simulink model "ModelSupervisor2"  (R2014b)
settings: Solver=ode3  StartTime=0.0  StopTime=T_max  FixedStep=h  RelTol=1e-3
values from neighbouring files (symbols this model uses):
  b = 0.1    [Input_LQR.m]    (also in TestKalman.m; TestSuper.m; TestVahidComparison.m; parameter.m)
  g = 9.81    [Input_LQR.m]    (also in TestKalman.m; TestSuper.m; TestVahidComparison.m; parameter.m = 9.8)
  h = 0.01    [Input_LQR.m]    (also in TestKalman.m = 0.001; TestSuper.m = 0.001; TestVahidComparison.m = 0.001; parameter.m)
  k = 0.15    [Input_LQR.m]    (also in TestKalman.m; TestSuper.m; TestVahidComparison.m; parameter.m)
  L = 1.4    [Input_LQR.m]    (also in TestKalman.m; TestSuper.m = 1.025; TestVahidComparison.m)
  M = 1    [Input_LQR.m]    (also in TestKalman.m; TestSuper.m; TestVahidComparison.m; parameter.m)
  m = 3/4    (= 0.75)    [Input_LQR.m]    (also in TestKalman.m; TestSuper.m; TestVahidComparison.m; parameter.m)
  theta_0 = 0    [Input_LQR.m]    (also in TestKalman.m = 0.1; TestSuper.m = 0.1; TestVahidComparison.m = 0.1)
  theta_dot0 = 0    [Input_LQR.m]    (also in TestKalman.m; TestSuper.m; TestVahidComparison.m)
  x_0 = 0    [Input_LQR.m]    (also in TestKalman.m; TestSuper.m; TestVahidComparison.m)
  x_dot0 = 0    [Input_LQR.m]    (also in TestKalman.m; TestSuper.m; TestVahidComparison.m)
undefined symbols (not defined in the file or in its folder): A_kA2, B_kA2, C_kA2, D_kA2
libraries: simulink x4
settings Model: Creator=Erik  LastModifiedBy=Erik
settings SolverCC: AlgebraicLoopSolver=LineSearch
settings OptimizationCC: UseDivisionForNetSlopeComputation=off  SimCompilerOptimization=off
settings DebuggingCC: FrameProcessingCompatibilityMsg=error
settings RTWCC: RTWCompilerOptimization=off
settings ConfigComp: CovMetricSettings=dw  CovHtmlReporting=on  CovSaveCumulativeToWorkspaceVar=on  CovSaveSingleToWorkspaceVar=on  CovModelRefEnable=Off  CovExternalEMLEnable=off  CovSFcnEnable=off

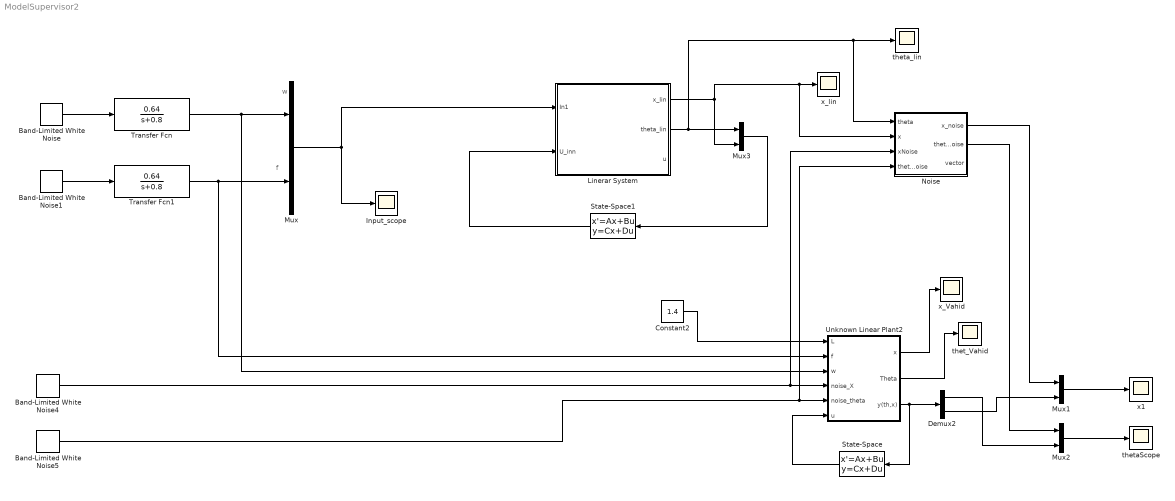
== system ModelSupervisor2 ==
  note: f
  note: w
  Band-Limited White Noise : simulink/Sources/Band-Limited White Noise  Cov=10  Ts=h  seed=[23343]
  Band-Limited White Noise1 : simulink/Sources/Band-Limited White Noise  Cov=10e-4  Ts=h  seed=[23344]
  Band-Limited White Noise4 : simulink/Sources/Band-Limited White Noise  Cov=10e-7  Ts=h  seed=[23343]
  Band-Limited White Noise5 : simulink/Sources/Band-Limited White Noise  Cov=10e-7  Ts=h  seed=[23344]
  Constant2 : Constant  Value=1.4
  Demux2 : Demux  Outputs=2
  Input_scope : Scope
      settings: YMin=-4  YMax=3  SaveName=ScopeData4
  Linerar System : Subsystem
  Mux{,1..3} (4 alike) : Mux  Inputs=2
  Noise : Subsystem
  State-Space : StateSpace  A=A_kA2  B=B_kA2  C=C_kA2  D=D_kA2  X0=0
  State-Space1 : StateSpace  A=A_kA2  B=B_kA2  C=C_kA2  D=D_kA2  X0=0
  Transfer Fcn : TransferFcn  Numerator=[0.64]  Denominator=[1 0.8]
  Transfer Fcn1 : TransferFcn  Numerator=[0.64]  Denominator=[1 0.8]
  Unknown Linear Plant2 : Subsystem
  thet_Vahid : Scope
      settings: SaveName=ScopeData3
  thetaScope : Scope
      settings: SaveName=ScopeData12
  theta_lin : Scope
      settings: YMin=-0.08  YMax=0.1  SaveName=ScopeData2
  x1 : Scope
      settings: YMin=-0.3  YMax=0.5  SaveName=ScopeData11
  x_Vahid : Scope
      settings: YMin=-0.15  YMax=0.1
  x_lin : Scope
      settings: YMin=-0.5  YMax=0.5
  wires:
  Mux/1 -> Linerar System/1(In1), Input_scope/1
  Band-Limited White Noise/1 -> Transfer Fcn/1
  Band-Limited White Noise1/1 -> Transfer Fcn1/1
  Linerar System/1(x_lin) -> Mux3/2, Noise/2(x), x_lin/1
  Unknown Linear Plant2/3(y(th,x)) -> Demux2/1, State-Space/1
  State-Space/1 -> Unknown Linear Plant2/6(u)
  Constant2/1 -> Unknown Linear Plant2/1(L)
  Demux2/1 -> Mux2/2
  Transfer Fcn/1 -> Mux/1, Unknown Linear Plant2/3(w)
  Transfer Fcn1/1 -> Unknown Linear Plant2/2(f), Mux/2
  Band-Limited White Noise4/1 -> Unknown Linear Plant2/4(noise_X), Noise/3(xNoise)
  Mux1/1 -> x1/1
  Mux2/1 -> thetaScope/1
  Linerar System/2(theta_lin) -> Mux3/1, Noise/1(theta), theta_lin/1
  Demux2/2 -> Mux1/2
  State-Space1/1 -> Linerar System/2(" U_inn")
  Mux3/1 -> State-Space1/1
  Noise/1(x_noise) -> Mux1/1
  Noise/2(theta_noise) -> Mux2/1
  Band-Limited White Noise5/1 -> Noise/4(thetaNoise), Unknown Linear Plant2/5(noise_theta)
  Unknown Linear Plant2/2(Theta) -> thet_Vahid/1
  Unknown Linear Plant2/1(x) -> x_Vahid/1

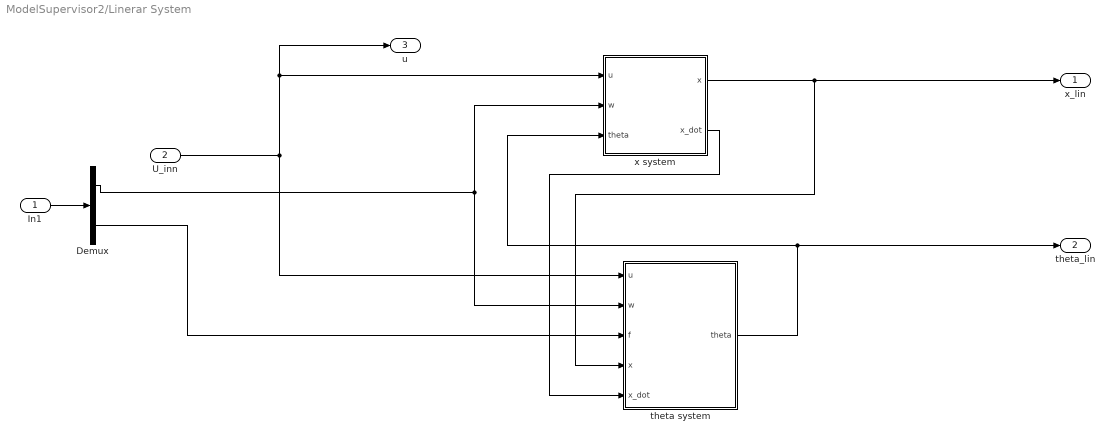
== system ModelSupervisor2/Linerar System ==
  In1 : Inport
  " U_inn" : Inport  Port=2
  Demux : Demux  Outputs=2
  "theta system " : Subsystem
  x system : Subsystem
  x_lin : Outport
  theta_lin : Outport  Port=2
  u : Outport  Port=3
  wires:
  x system/1(x) -> "theta system "/4(x), x_lin/1
  Demux/1 -> "theta system "/2(w), x system/2(w)
  "theta system "/1(theta) -> theta_lin/1, x system/3(theta)
  Demux/2 -> "theta system "/3(f)
  x system/2(x_dot) -> "theta system "/5(x_dot)
  In1/1 -> Demux/1
  " U_inn"/1 -> u/1, x system/1("u "), "theta system "/1("u ")

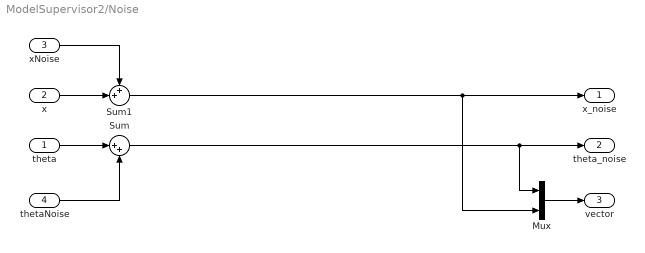
== system ModelSupervisor2/Noise ==
  theta : Inport
  x : Inport  Port=2
  xNoise : Inport  Port=3
  thetaNoise : Inport  Port=4
  Mux : Mux  Inputs=2
  Sum : Sum  Inputs=|++
  Sum1 : Sum  Inputs=++|
  x_noise : Outport
  theta_noise : Outport  Port=2
  vector : Outport  Port=3
  wires:
  xNoise/1 -> Sum1/1
  x/1 -> Sum1/2
  theta/1 -> Sum/1
  thetaNoise/1 -> Sum/2
  Sum/1 -> Mux/1, theta_noise/1
  Mux/1 -> vector/1
  Sum1/1 -> Mux/2, x_noise/1

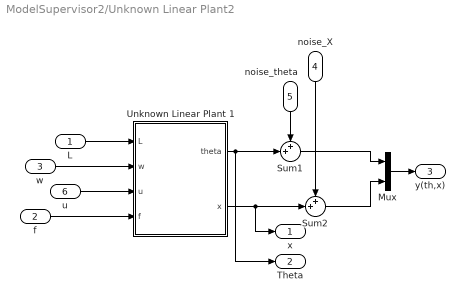
== system ModelSupervisor2/Unknown Linear Plant2 ==
  L : Inport
  f : Inport  Port=2
  w : Inport  Port=3
  noise_X : Inport  Port=4
  noise_theta : Inport  Port=5
  u : Inport  Port=6
  Mux : Mux  Inputs=2
  Sum1 : Sum  Inputs=++|
  Sum2 : Sum  Inputs=++|
  Unknown Linear Plant 1 : Subsystem
  x : Outport
  Theta : Outport  Port=2
  y(th,x) : Outport  Port=3
  wires:
  Mux/1 -> y(th,x)/1
  Sum2/1 -> Mux/2
  Sum1/1 -> Mux/1
  noise_X/1 -> Sum2/1
  Unknown Linear Plant 1/2(x) -> x/1, Sum2/2
  noise_theta/1 -> Sum1/1
  Unknown Linear Plant 1/1(theta) -> Theta/1, Sum1/2
  w/1 -> Unknown Linear Plant 1/2(w)
  L/1 -> Unknown Linear Plant 1/1(L)
  u/1 -> Unknown Linear Plant 1/3(u)
  f/1 -> Unknown Linear Plant 1/4(f)

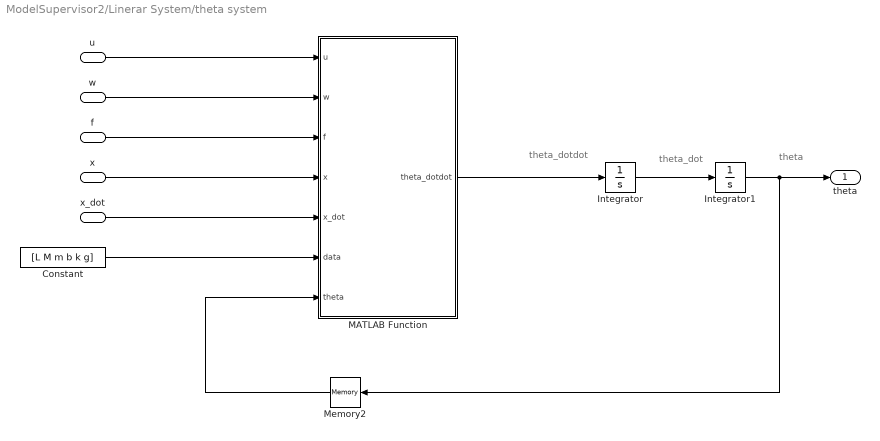
== system ModelSupervisor2/Linerar System/theta system  ==
  note: theta
  note: theta_dotdot
  note: theta_dot
  "u " : Inport
  w : Inport  Port=2
  f : Inport  Port=3
  x : Inport  Port=4
  x_dot : Inport  Port=5
  Constant : Constant  Value=[L M m b k g]  VectorParams1D=off  SampleTime=0.01
  Integrator : Integrator  InitialCondition=theta_dot0
  Integrator1 : Integrator  InitialCondition=theta_0
  MATLAB Function : MATLAB Function  TreatAsAtomicUnit=on
  Memory2 : Memory  X0=theta_0
  theta : Outport
  wires:
  MATLAB Function/1(theta_dotdot) -> Integrator/1
  "u "/1 -> MATLAB Function/1(u)
  w/1 -> MATLAB Function/2(w)
  x/1 -> MATLAB Function/4(x)
  Integrator1/1 -> Memory2/1, theta/1
  Constant/1 -> MATLAB Function/6(data)
  f/1 -> MATLAB Function/3(f)
  x_dot/1 -> MATLAB Function/5(x_dot)
  Memory2/1 -> MATLAB Function/7(theta)
  Integrator/1 -> Integrator1/1

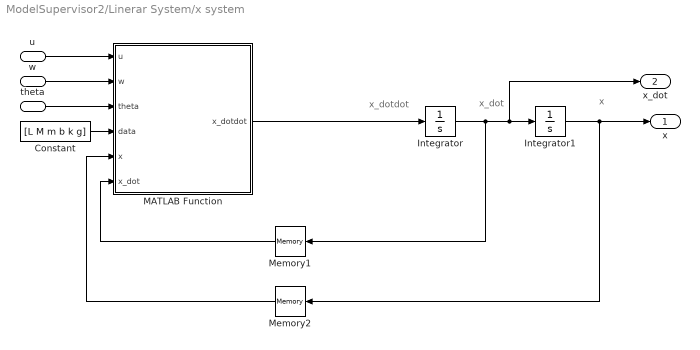
== system ModelSupervisor2/Linerar System/x system ==
  note: x
  note: x_dotdot
  note: x_dot
  "u " : Inport
  w : Inport  Port=2
  theta : Inport  Port=3
  Constant : Constant  Value=[L M m b k g]  VectorParams1D=off  SampleTime=0.01
  Integrator : Integrator  InitialCondition=x_dot0
  Integrator1 : Integrator  InitialCondition=x_0
  MATLAB Function : MATLAB Function  TreatAsAtomicUnit=on
  Memory1 : Memory  X0=x_dot0
  Memory2 : Memory  X0=x_0
  x : Outport
  x_dot : Outport  Port=2
  wires:
  Memory1/1 -> MATLAB Function/6(x_dot)
  "u "/1 -> MATLAB Function/1(u)
  w/1 -> MATLAB Function/2(w)
  theta/1 -> MATLAB Function/3(theta)
  Integrator1/1 -> Memory2/1, x/1
  Memory2/1 -> MATLAB Function/5(x)
  Constant/1 -> MATLAB Function/4(data)
  Integrator/1 -> Integrator1/1, x_dot/1, Memory1/1
  MATLAB Function/1(x_dotdot) -> Integrator/1

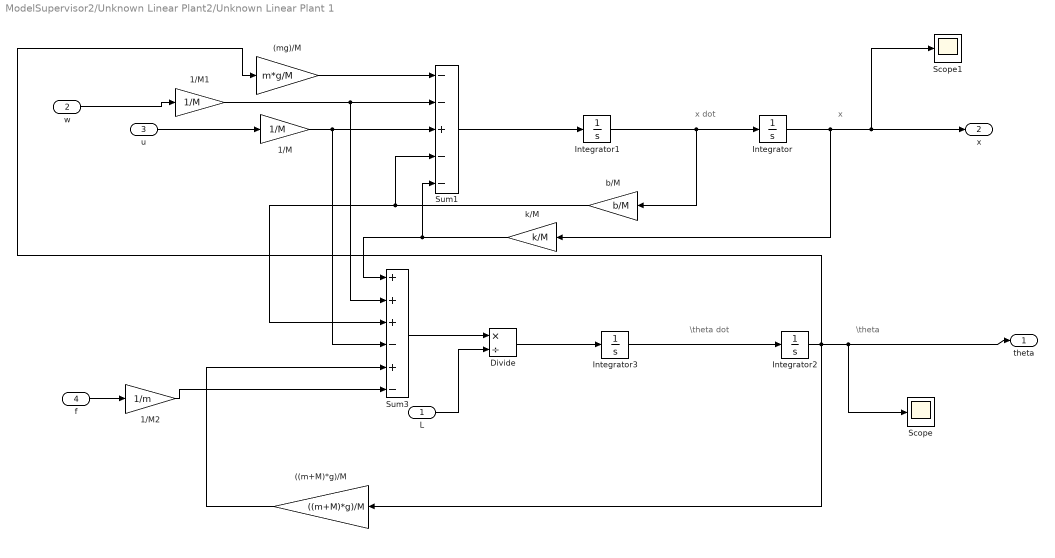
== system ModelSupervisor2/Unknown Linear Plant2/Unknown Linear Plant 1 ==
  note: \theta dot
  note: x dot
  note: \theta
  note: x
  L : Inport
  w : Inport  Port=2
  u : Inport  Port=3
  f : Inport  Port=4
  ((m+M)*g)/M : Gain  Gain=((m+M)*g)/M
  (mg)/M : Gain  Gain=m*g/M
  1/M : Gain  Gain=1/M
  1/M1 : Gain  Gain=1/M
  1/M2 : Gain  Gain=1/m
  Divide : Product  Inputs=*/
  Integrator{,1..3} (4 alike) : Integrator
  Scope : Scope
      settings: YMin=0  YMax=32.5  SaveName=ScopeData4
  Scope1 : Scope
      settings: YMin=0.12  YMax=0.175  SaveName=ScopeData5
  Sum1 : Sum  Inputs=--+--
  Sum3 : Sum  Inputs=+++-+-
  b/M : Gain  Gain=b/M
  k/M : Gain  Gain=k/M
  theta : Outport
  x : Outport  Port=2
  wires:
  k/M/1 -> Sum3/1, Sum1/5
  Integrator3/1 -> Integrator2/1
  Integrator1/1 -> Integrator/1, b/M/1
  Integrator/1 -> k/M/1, Scope1/1, x/1
  Integrator2/1 -> Scope/1, theta/1, (mg)/M/1, ((m+M)*g)/M/1
  u/1 -> 1/M/1
  b/M/1 -> Sum3/3, Sum1/4
  1/M/1 -> Sum3/4, Sum1/3
  w/1 -> 1/M1/1
  1/M1/1 -> Sum3/2, Sum1/2
  (mg)/M/1 -> Sum1/1
  Sum1/1 -> Integrator1/1
  Sum3/1 -> Divide/1
  Divide/1 -> Integrator3/1
  L/1 -> Divide/2
  ((m+M)*g)/M/1 -> Sum3/5
  f/1 -> 1/M2/1
  1/M2/1 -> Sum3/6

== matlab function ModelSupervisor2/Linerar System/x system/MATLAB Function ==
  data: u input; w input; theta input; data input; x_dotdot output; x input; x_dot input
function x_dotdot  = fcn(u, w, theta, data, x, x_dot)
L = data(1);
M = data(2);
m = data(3);
b = data(4);
k = data(5);
g = data(6);

% theta = theta * 180 / pi;

x_dotdot=(u - w - m * g * theta - b * x_dot - k * x) / M;


end

== matlab function ModelSupervisor2/Linerar System/theta system /MATLAB Function ==
  data: u input; w input; f input; x input; x_dot input; data input; theta input; theta_dotdot output
function theta_dotdot  = fcn(u, w, f, x, x_dot, data, theta)
L = data(1);
M = data(2);
m = data(3);
b = data(4);
k = data(5);
g = data(6);

% theta = theta * 180 / pi;

theta_dotdot=(-u + w + (m + M) * g * theta - (M / m) * f + b * x_dot + k * x)/(L * M);

end
